simulink model "Passive_BMS"  (R2024b)
settings: Solver=FixedStepDiscrete  StartTime=0.0  StopTime=0.1  FixedStep=0.01  MaxStep=0.1  RelTol=1e-3
undefined symbols (not defined in the file): DiscIntNeverNeededParam
settings Model: Creator=rakes  LastModifiedBy=rakes

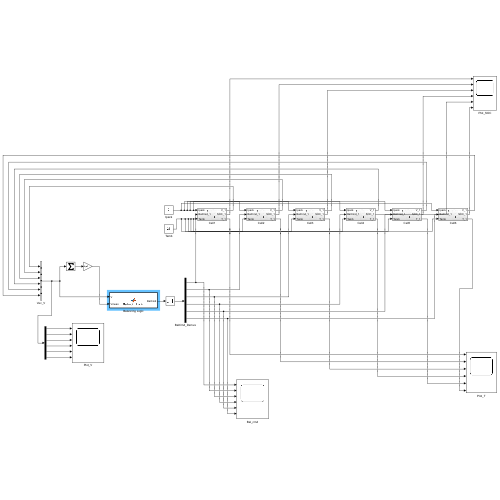
[thumbnail: Simulink's stored preview of the top-level diagram]
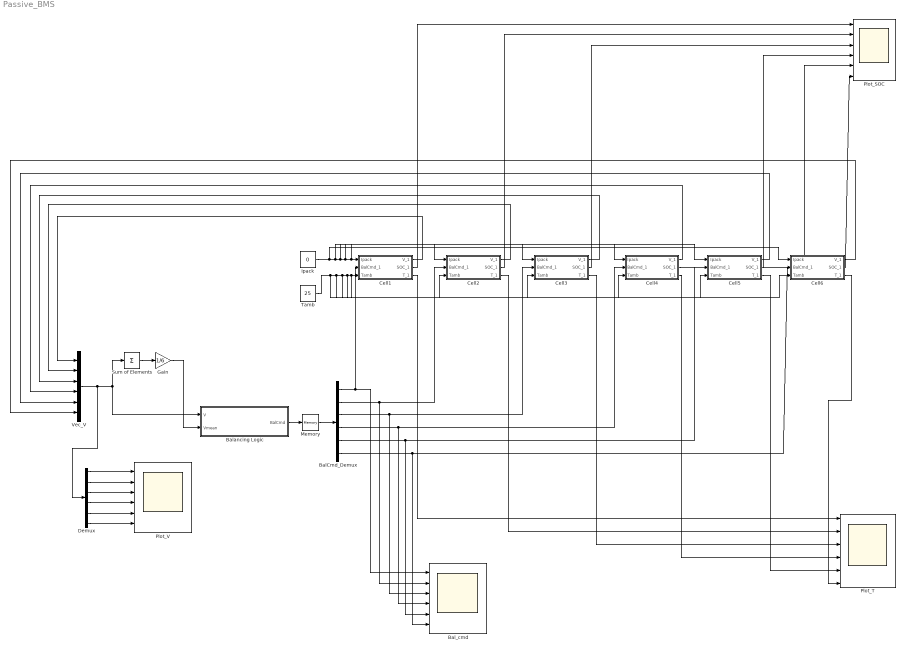
== system Passive_BMS ==
  BalCmd_Demux : Demux  Outputs=6
  Bal_cmd : Scope  NumInputPorts=6
  Balancing Logic : MATLAB Function  TreatAsAtomicUnit=on  SystemSampleTime=0.01
  Cell1 : Subsystem
  Cell2 : Subsystem
  Cell3 : Subsystem
  Cell4 : Subsystem
  Cell5 : Subsystem
  Cell6 : Subsystem
  Demux : Demux  Outputs=6
  Gain : Gain  Gain=1/6
  Ipack : Constant  Value=0
  Memory : Memory  InheritSampleTime=on
  Plot_SOC : Scope  NumInputPorts=6
  Plot_T : Scope  NumInputPorts=6
  Plot_V : Scope  NumInputPorts=6
  Sum of Elements : Sum  Inputs=+
  Tamb : Constant  Value=25
  Vec_V : Concatenate  NumInputs=6
  wires:
  Ipack/1 -> Cell6/1(Ipack), Cell5/1(Ipack), Cell4/1(Ipack), Cell3/1(Ipack), Cell2/1(Ipack), Cell1/1(Ipack)
  Tamb/1 -> Cell6/3(Tamb), Cell5/3(Tamb), Cell4/3(Tamb), Cell3/3(Tamb), Cell2/3(Tamb), Cell1/3(Tamb)
  Vec_V/1 -> Demux/1, Sum of Elements/1, Balancing Logic/1(V)
  Gain/1 -> Balancing Logic/2(Vmean)
  BalCmd_Demux/1 -> Bal_cmd/1, Cell1/2(BalCmd_1)
  BalCmd_Demux/2 -> Bal_cmd/2, Cell2/2(BalCmd_1)
  BalCmd_Demux/3 -> Bal_cmd/3, Cell3/2(BalCmd_1)
  BalCmd_Demux/4 -> Bal_cmd/4, Cell4/2(BalCmd_1)
  BalCmd_Demux/5 -> Bal_cmd/5, Cell5/2(BalCmd_1)
  BalCmd_Demux/6 -> Bal_cmd/6, Cell6/2(BalCmd_1)
  Cell1/1(V_1) -> Vec_V/1
  Cell2/1(V_1) -> Vec_V/2
  Cell3/1(V_1) -> Vec_V/3
  Cell4/1(V_1) -> Vec_V/4
  Cell5/1(V_1) -> Vec_V/5
  Cell6/1(V_1) -> Vec_V/6
  Cell1/3(T_1) -> Plot_T/1
  Cell2/3(T_1) -> Plot_T/2
  Cell3/3(T_1) -> Plot_T/3
  Cell4/3(T_1) -> Plot_T/4
  Cell5/3(T_1) -> Plot_T/5
  Cell6/3(T_1) -> Plot_T/6
  Cell1/2(SOC_1) -> Plot_SOC/1
  Cell2/2(SOC_1) -> Plot_SOC/2
  Cell3/2(SOC_1) -> Plot_SOC/3
  Cell4/2(SOC_1) -> Plot_SOC/4
  Cell5/2(SOC_1) -> Plot_SOC/5
  Cell6/2(SOC_1) -> Plot_SOC/6
  Balancing Logic/1(BalCmd) -> Memory/1
  Memory/1 -> BalCmd_Demux/1
  Sum of Elements/1 -> Gain/1
  Demux/1 -> Plot_V/1
  Demux/2 -> Plot_V/2
  Demux/3 -> Plot_V/3
  Demux/4 -> Plot_V/4
  Demux/5 -> Plot_V/5
  Demux/6 -> Plot_V/6

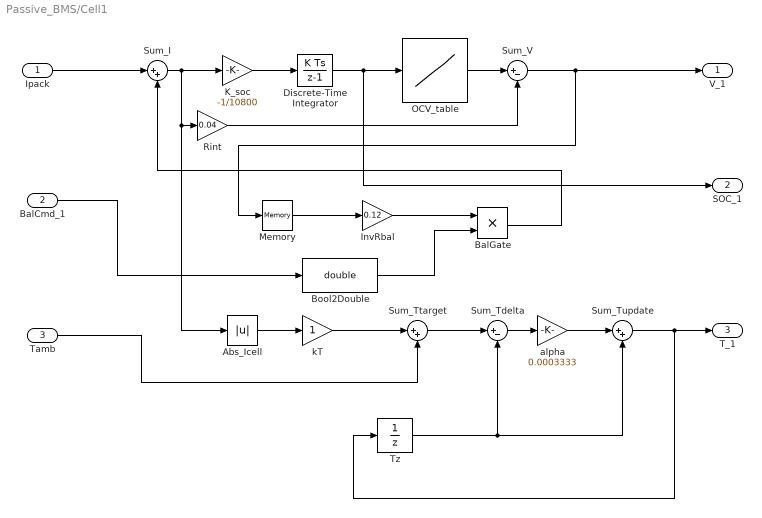
== system Passive_BMS/Cell1 ==
  Ipack : Inport
  BalCmd_1 : Inport  Port=2
  Tamb : Inport  Port=3
  Abs_Icell : Abs  SaturateOnIntegerOverflow=off
  BalGate : Product
  Bool2Double : DataTypeConversion  OutDataTypeStr=double  SaturateOnIntegerOverflow=off  RndMeth=Floor
  Discrete-Time Integrator : DiscreteIntegrator  gainval=1  InitialCondition=0.82  SampleTime=0.01  LimitOutput=on  UpperSaturationLimit=1  LowerSaturationLimit=0  ICPrevOutput=DiscIntNeverNeededParam  ICPrevScaledInput=DiscIntNeverNeededParam
  InvRbal : Gain  Gain=0.12
  K_soc : Gain  Gain=-1/10800
  Memory : Memory  InitialCondition=3.8
  OCV_table : Lookup_n-D  NumberOfTableDimensions=1  BreakpointsForDimension1=[0 0.1 0.2 0.4 0.6 0.8 0.9 1]  Table=[3.0 3.4 3.55 3.75 3.90 4.00 4.08 4.20]  InternalRulePriority=Speed  RndMeth=Simplest
  Rint : Gain  Gain=0.04
  Sum_I : Sum  Inputs=|++
  Sum_Tdelta : Sum  Inputs=|+-
  Sum_Ttarget : Sum  Inputs=|++
  Sum_Tupdate : Sum  Inputs=|++
  Sum_V : Sum  Inputs=|+-
  Tz : UnitDelay  InitialCondition=25  SampleTime=-1  HasFrameUpgradeWarning=on
  alpha : Gain  Gain=0.0003333
  kT : Gain
  V_1 : Outport
  SOC_1 : Outport  Port=2
  T_1 : Outport  Port=3
  wires:
  Ipack/1 -> Sum_I/1
  Memory/1 -> InvRbal/1
  BalCmd_1/1 -> Bool2Double/1
  Bool2Double/1 -> BalGate/2
  InvRbal/1 -> BalGate/1
  BalGate/1 -> Sum_I/2
  Sum_I/1 -> Abs_Icell/1, Rint/1, K_soc/1
  K_soc/1 -> Discrete-Time Integrator/1
  Discrete-Time Integrator/1 -> SOC_1/1, OCV_table/1
  OCV_table/1 -> Sum_V/1
  Rint/1 -> Sum_V/2
  Sum_V/1 -> Memory/1, V_1/1
  Abs_Icell/1 -> kT/1
  kT/1 -> Sum_Ttarget/1
  Tamb/1 -> Sum_Ttarget/2
  Sum_Ttarget/1 -> Sum_Tdelta/1
  Tz/1 -> Sum_Tupdate/2, Sum_Tdelta/2
  Sum_Tdelta/1 -> alpha/1
  alpha/1 -> Sum_Tupdate/1
  Sum_Tupdate/1 -> T_1/1, Tz/1

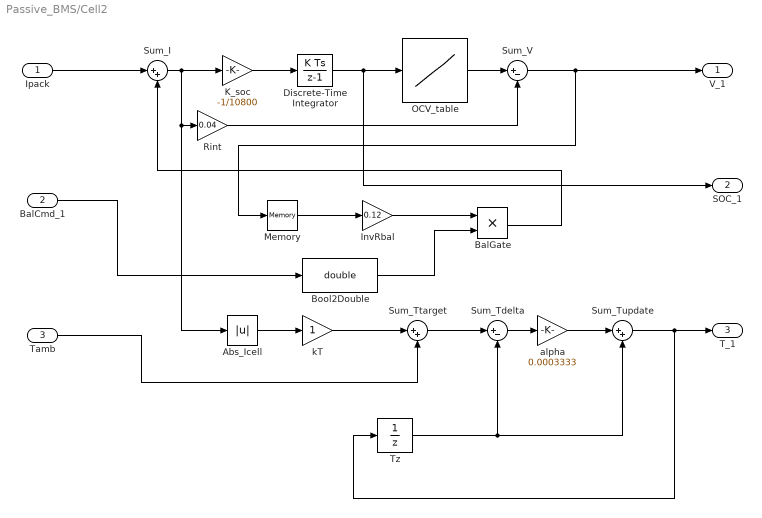
== system Passive_BMS/Cell2 ==
  Ipack : Inport
  BalCmd_1 : Inport  Port=2
  Tamb : Inport  Port=3
  Abs_Icell : Abs  SaturateOnIntegerOverflow=off
  BalGate : Product
  Bool2Double : DataTypeConversion  OutDataTypeStr=double  SaturateOnIntegerOverflow=off  RndMeth=Floor
  Discrete-Time Integrator : DiscreteIntegrator  gainval=1  InitialCondition=0.76  SampleTime=0.01  LimitOutput=on  UpperSaturationLimit=1  LowerSaturationLimit=0  ICPrevOutput=DiscIntNeverNeededParam  ICPrevScaledInput=DiscIntNeverNeededParam
  InvRbal : Gain  Gain=0.12
  K_soc : Gain  Gain=-1/10800
  Memory : Memory  InitialCondition=3.8
  OCV_table : Lookup_n-D  NumberOfTableDimensions=1  BreakpointsForDimension1=[0 0.1 0.2 0.4 0.6 0.8 0.9 1]  Table=[3.0 3.4 3.55 3.75 3.90 4.00 4.08 4.20]  InternalRulePriority=Speed  RndMeth=Simplest
  Rint : Gain  Gain=0.04
  Sum_I : Sum  Inputs=|++
  Sum_Tdelta : Sum  Inputs=|+-
  Sum_Ttarget : Sum  Inputs=|++
  Sum_Tupdate : Sum  Inputs=|++
  Sum_V : Sum  Inputs=|+-
  Tz : UnitDelay  InitialCondition=25  SampleTime=-1  HasFrameUpgradeWarning=on
  alpha : Gain  Gain=0.0003333
  kT : Gain
  V_1 : Outport
  SOC_1 : Outport  Port=2
  T_1 : Outport  Port=3
  wires:
  Ipack/1 -> Sum_I/1
  Memory/1 -> InvRbal/1
  BalCmd_1/1 -> Bool2Double/1
  Bool2Double/1 -> BalGate/2
  InvRbal/1 -> BalGate/1
  BalGate/1 -> Sum_I/2
  Sum_I/1 -> Abs_Icell/1, Rint/1, K_soc/1
  K_soc/1 -> Discrete-Time Integrator/1
  Discrete-Time Integrator/1 -> SOC_1/1, OCV_table/1
  OCV_table/1 -> Sum_V/1
  Rint/1 -> Sum_V/2
  Sum_V/1 -> Memory/1, V_1/1
  Abs_Icell/1 -> kT/1
  kT/1 -> Sum_Ttarget/1
  Tamb/1 -> Sum_Ttarget/2
  Sum_Ttarget/1 -> Sum_Tdelta/1
  Tz/1 -> Sum_Tupdate/2, Sum_Tdelta/2
  Sum_Tdelta/1 -> alpha/1
  alpha/1 -> Sum_Tupdate/1
  Sum_Tupdate/1 -> T_1/1, Tz/1

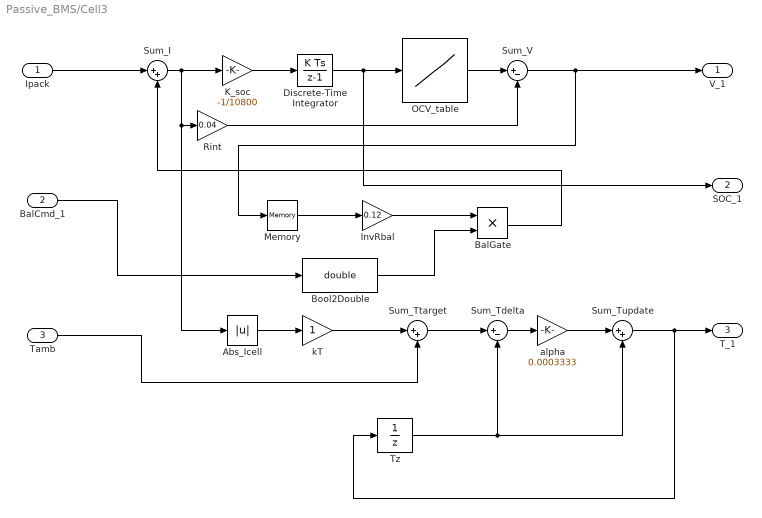
== system Passive_BMS/Cell3 ==
  Ipack : Inport
  BalCmd_1 : Inport  Port=2
  Tamb : Inport  Port=3
  Abs_Icell : Abs  SaturateOnIntegerOverflow=off
  BalGate : Product
  Bool2Double : DataTypeConversion  OutDataTypeStr=double  SaturateOnIntegerOverflow=off  RndMeth=Floor
  Discrete-Time Integrator : DiscreteIntegrator  gainval=1  InitialCondition=0.80  SampleTime=0.01  LimitOutput=on  UpperSaturationLimit=1  LowerSaturationLimit=0  ICPrevOutput=DiscIntNeverNeededParam  ICPrevScaledInput=DiscIntNeverNeededParam
  InvRbal : Gain  Gain=0.12
  K_soc : Gain  Gain=-1/10800
  Memory : Memory  InitialCondition=3.8
  OCV_table : Lookup_n-D  NumberOfTableDimensions=1  BreakpointsForDimension1=[0 0.1 0.2 0.4 0.6 0.8 0.9 1]  Table=[3.0 3.4 3.55 3.75 3.90 4.00 4.08 4.20]  InternalRulePriority=Speed  RndMeth=Simplest
  Rint : Gain  Gain=0.04
  Sum_I : Sum  Inputs=|++
  Sum_Tdelta : Sum  Inputs=|+-
  Sum_Ttarget : Sum  Inputs=|++
  Sum_Tupdate : Sum  Inputs=|++
  Sum_V : Sum  Inputs=|+-
  Tz : UnitDelay  InitialCondition=25  SampleTime=-1  HasFrameUpgradeWarning=on
  alpha : Gain  Gain=0.0003333
  kT : Gain
  V_1 : Outport
  SOC_1 : Outport  Port=2
  T_1 : Outport  Port=3
  wires:
  Ipack/1 -> Sum_I/1
  Memory/1 -> InvRbal/1
  BalCmd_1/1 -> Bool2Double/1
  Bool2Double/1 -> BalGate/2
  InvRbal/1 -> BalGate/1
  BalGate/1 -> Sum_I/2
  Sum_I/1 -> Abs_Icell/1, Rint/1, K_soc/1
  K_soc/1 -> Discrete-Time Integrator/1
  Discrete-Time Integrator/1 -> SOC_1/1, OCV_table/1
  OCV_table/1 -> Sum_V/1
  Rint/1 -> Sum_V/2
  Sum_V/1 -> Memory/1, V_1/1
  Abs_Icell/1 -> kT/1
  kT/1 -> Sum_Ttarget/1
  Tamb/1 -> Sum_Ttarget/2
  Sum_Ttarget/1 -> Sum_Tdelta/1
  Tz/1 -> Sum_Tupdate/2, Sum_Tdelta/2
  Sum_Tdelta/1 -> alpha/1
  alpha/1 -> Sum_Tupdate/1
  Sum_Tupdate/1 -> T_1/1, Tz/1

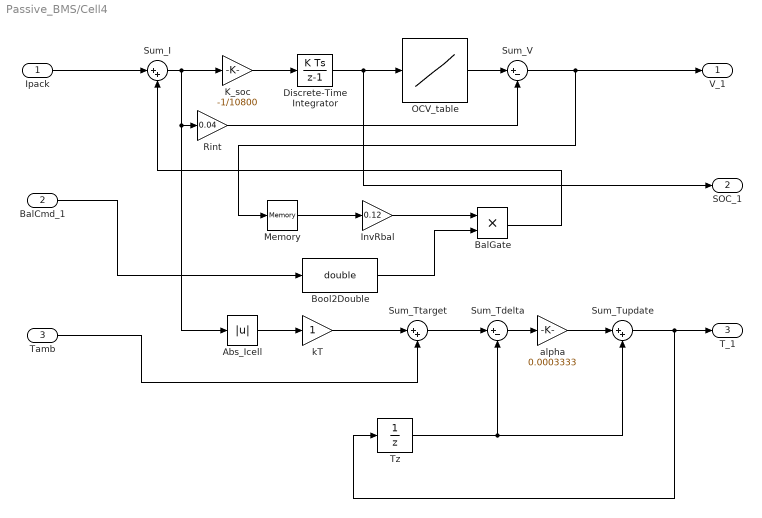
== system Passive_BMS/Cell4 ==
  Ipack : Inport
  BalCmd_1 : Inport  Port=2
  Tamb : Inport  Port=3
  Abs_Icell : Abs  SaturateOnIntegerOverflow=off
  BalGate : Product
  Bool2Double : DataTypeConversion  OutDataTypeStr=double  SaturateOnIntegerOverflow=off  RndMeth=Floor
  Discrete-Time Integrator : DiscreteIntegrator  gainval=1  InitialCondition=0.79  SampleTime=0.01  LimitOutput=on  UpperSaturationLimit=1  LowerSaturationLimit=0  ICPrevOutput=DiscIntNeverNeededParam  ICPrevScaledInput=DiscIntNeverNeededParam
  InvRbal : Gain  Gain=0.12
  K_soc : Gain  Gain=-1/10800
  Memory : Memory  InitialCondition=3.8
  OCV_table : Lookup_n-D  NumberOfTableDimensions=1  BreakpointsForDimension1=[0 0.1 0.2 0.4 0.6 0.8 0.9 1]  Table=[3.0 3.4 3.55 3.75 3.90 4.00 4.08 4.20]  InternalRulePriority=Speed  RndMeth=Simplest
  Rint : Gain  Gain=0.04
  Sum_I : Sum  Inputs=|++
  Sum_Tdelta : Sum  Inputs=|+-
  Sum_Ttarget : Sum  Inputs=|++
  Sum_Tupdate : Sum  Inputs=|++
  Sum_V : Sum  Inputs=|+-
  Tz : UnitDelay  InitialCondition=25  SampleTime=-1  HasFrameUpgradeWarning=on
  alpha : Gain  Gain=0.0003333
  kT : Gain
  V_1 : Outport
  SOC_1 : Outport  Port=2
  T_1 : Outport  Port=3
  wires:
  Ipack/1 -> Sum_I/1
  Memory/1 -> InvRbal/1
  BalCmd_1/1 -> Bool2Double/1
  Bool2Double/1 -> BalGate/2
  InvRbal/1 -> BalGate/1
  BalGate/1 -> Sum_I/2
  Sum_I/1 -> Abs_Icell/1, Rint/1, K_soc/1
  K_soc/1 -> Discrete-Time Integrator/1
  Discrete-Time Integrator/1 -> SOC_1/1, OCV_table/1
  OCV_table/1 -> Sum_V/1
  Rint/1 -> Sum_V/2
  Sum_V/1 -> Memory/1, V_1/1
  Abs_Icell/1 -> kT/1
  kT/1 -> Sum_Ttarget/1
  Tamb/1 -> Sum_Ttarget/2
  Sum_Ttarget/1 -> Sum_Tdelta/1
  Tz/1 -> Sum_Tupdate/2, Sum_Tdelta/2
  Sum_Tdelta/1 -> alpha/1
  alpha/1 -> Sum_Tupdate/1
  Sum_Tupdate/1 -> T_1/1, Tz/1

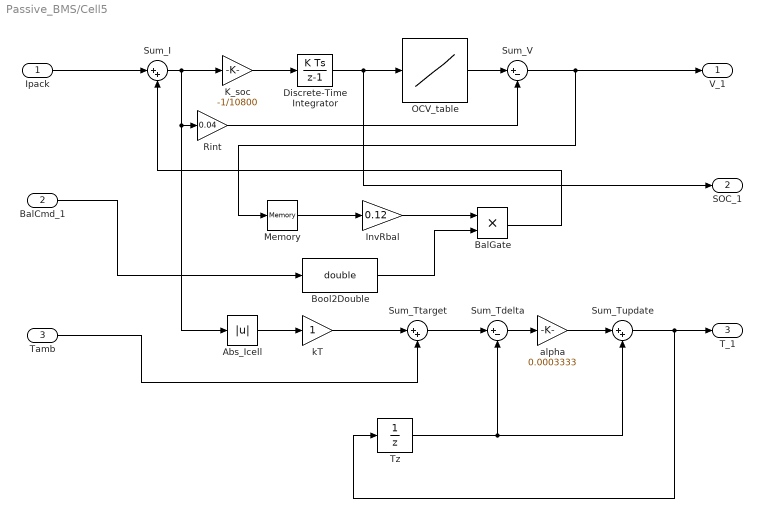
== system Passive_BMS/Cell5 ==
  Ipack : Inport
  BalCmd_1 : Inport  Port=2
  Tamb : Inport  Port=3
  Abs_Icell : Abs  SaturateOnIntegerOverflow=off
  BalGate : Product
  Bool2Double : DataTypeConversion  OutDataTypeStr=double  SaturateOnIntegerOverflow=off  RndMeth=Floor
  Discrete-Time Integrator : DiscreteIntegrator  gainval=1  InitialCondition=0.83  SampleTime=0.01  LimitOutput=on  UpperSaturationLimit=1  LowerSaturationLimit=0  ICPrevOutput=DiscIntNeverNeededParam  ICPrevScaledInput=DiscIntNeverNeededParam
  InvRbal : Gain  Gain=0.12
  K_soc : Gain  Gain=-1/10800
  Memory : Memory  InitialCondition=3.8
  OCV_table : Lookup_n-D  NumberOfTableDimensions=1  BreakpointsForDimension1=[0 0.1 0.2 0.4 0.6 0.8 0.9 1]  Table=[3.0 3.4 3.55 3.75 3.90 4.00 4.08 4.20]  InternalRulePriority=Speed  RndMeth=Simplest
  Rint : Gain  Gain=0.04
  Sum_I : Sum  Inputs=|++
  Sum_Tdelta : Sum  Inputs=|+-
  Sum_Ttarget : Sum  Inputs=|++
  Sum_Tupdate : Sum  Inputs=|++
  Sum_V : Sum  Inputs=|+-
  Tz : UnitDelay  InitialCondition=25  SampleTime=-1  HasFrameUpgradeWarning=on
  alpha : Gain  Gain=0.0003333
  kT : Gain
  V_1 : Outport
  SOC_1 : Outport  Port=2
  T_1 : Outport  Port=3
  wires:
  Ipack/1 -> Sum_I/1
  Memory/1 -> InvRbal/1
  BalCmd_1/1 -> Bool2Double/1
  Bool2Double/1 -> BalGate/2
  InvRbal/1 -> BalGate/1
  BalGate/1 -> Sum_I/2
  Sum_I/1 -> Abs_Icell/1, Rint/1, K_soc/1
  K_soc/1 -> Discrete-Time Integrator/1
  Discrete-Time Integrator/1 -> SOC_1/1, OCV_table/1
  OCV_table/1 -> Sum_V/1
  Rint/1 -> Sum_V/2
  Sum_V/1 -> Memory/1, V_1/1
  Abs_Icell/1 -> kT/1
  kT/1 -> Sum_Ttarget/1
  Tamb/1 -> Sum_Ttarget/2
  Sum_Ttarget/1 -> Sum_Tdelta/1
  Tz/1 -> Sum_Tupdate/2, Sum_Tdelta/2
  Sum_Tdelta/1 -> alpha/1
  alpha/1 -> Sum_Tupdate/1
  Sum_Tupdate/1 -> T_1/1, Tz/1

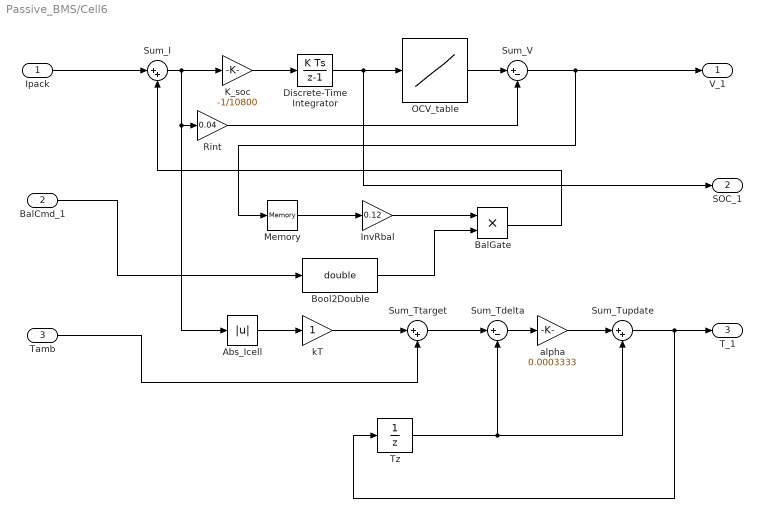
== system Passive_BMS/Cell6 ==
  Ipack : Inport
  BalCmd_1 : Inport  Port=2
  Tamb : Inport  Port=3
  Abs_Icell : Abs  SaturateOnIntegerOverflow=off
  BalGate : Product
  Bool2Double : DataTypeConversion  OutDataTypeStr=double  SaturateOnIntegerOverflow=off  RndMeth=Floor
  Discrete-Time Integrator : DiscreteIntegrator  gainval=1  InitialCondition=0.78  SampleTime=0.01  LimitOutput=on  UpperSaturationLimit=1  LowerSaturationLimit=0  ICPrevOutput=DiscIntNeverNeededParam  ICPrevScaledInput=DiscIntNeverNeededParam
  InvRbal : Gain  Gain=0.12
  K_soc : Gain  Gain=-1/10800
  Memory : Memory  InitialCondition=3.8
  OCV_table : Lookup_n-D  NumberOfTableDimensions=1  BreakpointsForDimension1=[0 0.1 0.2 0.4 0.6 0.8 0.9 1]  Table=[3.0 3.4 3.55 3.75 3.90 4.00 4.08 4.20]  InternalRulePriority=Speed  RndMeth=Simplest
  Rint : Gain  Gain=0.04
  Sum_I : Sum  Inputs=|++
  Sum_Tdelta : Sum  Inputs=|+-
  Sum_Ttarget : Sum  Inputs=|++
  Sum_Tupdate : Sum  Inputs=|++
  Sum_V : Sum  Inputs=|+-
  Tz : UnitDelay  InitialCondition=25  SampleTime=-1  HasFrameUpgradeWarning=on
  alpha : Gain  Gain=0.0003333
  kT : Gain
  V_1 : Outport
  SOC_1 : Outport  Port=2
  T_1 : Outport  Port=3
  wires:
  Ipack/1 -> Sum_I/1
  Memory/1 -> InvRbal/1
  BalCmd_1/1 -> Bool2Double/1
  Bool2Double/1 -> BalGate/2
  InvRbal/1 -> BalGate/1
  BalGate/1 -> Sum_I/2
  Sum_I/1 -> Abs_Icell/1, Rint/1, K_soc/1
  K_soc/1 -> Discrete-Time Integrator/1
  Discrete-Time Integrator/1 -> SOC_1/1, OCV_table/1
  OCV_table/1 -> Sum_V/1
  Rint/1 -> Sum_V/2
  Sum_V/1 -> Memory/1, V_1/1
  Abs_Icell/1 -> kT/1
  kT/1 -> Sum_Ttarget/1
  Tamb/1 -> Sum_Ttarget/2
  Sum_Ttarget/1 -> Sum_Tdelta/1
  Tz/1 -> Sum_Tupdate/2, Sum_Tdelta/2
  Sum_Tdelta/1 -> alpha/1
  alpha/1 -> Sum_Tupdate/1
  Sum_Tupdate/1 -> T_1/1, Tz/1

== matlab function Passive_BMS/Balancing Logic ==
  data: V input; BalCmd output; Vmean input
function BalCmd = BalancingLogic(V, Vmean)
% V: 1x6 vector of cell voltages
% Vmean: scalar mean (guard if vector)
Vmean = Vmean(1);

% Hysteresis thresholds
dV_on  = 0.003;   % 3 mV to turn ON
dV_off = 0.001;   % 1 mV to turn OFF (smaller than ON)

persistent state
if isempty(state)
    state = false(size(V));  % one state bit per cell
end

for i = 1:numel(V)
    if state(i)
        % keep ON until the cell falls well below the mean
        state(i) = V(i) > Vmean + dV_off;
    else
        % only start when clearly high
        state(i) = V(i) > Vmean + dV_on;
    end
end

BalCmd = state;
end
